simulink model "parameter_estimation"  (R2016a)
settings: Solver=VariableStepAuto  StartTime=0.0  StopTime=10.0  RelTol=1e-3
model workspace (MAT data in the model file):
  parameter_estimation_spesession : sldodialogs.data.SessionData (value not decoded)
undefined symbols (not defined in the file): Ts
settings Model: Creator=User  LastModifiedBy=User

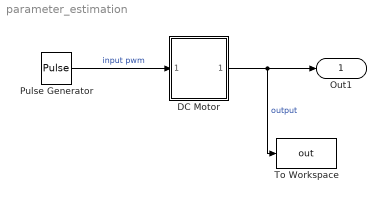
== system parameter_estimation ==
  DC Motor : Subsystem  mask(DC Motor){b=0.272617645619831, J=0.010032184368255, K=0.036496812786540, R=0.233319374033541, L=0.010005916298972}
      mask prompts: b "Damping:"; J "Inertia:"; K "Back EMF:"; R "Resistance:"; L "Inductance:"
      mask help: An ideal model of a DC Motor
      mask Help: This is <b>more elaborate<b> help.
      mask Display: image(imread('dcmotor.jpg'))
  Pulse Generator : DiscretePulseGenerator  PulseType=Time based  Period=0.1  PulseWidth=50  SampleTime=Ts  VectorParams1D=off
  To Workspace : ToWorkspace  VariableName=out  SampleTime=-1
  Out1 : Outport
  wires:
  DC Motor/1(Speed) -> To Workspace/1, Out1/1  "output"
  Pulse Generator/1 -> DC Motor/1(Voltage)  "input pwm"

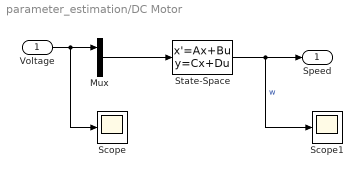
== system parameter_estimation/DC Motor ==
  Voltage : Inport
  Mux : Mux  Inputs=2
  Scope : Scope
  Scope1 : Scope
  State-Space : StateSpace  A=[-b/J K/J; -K/L -R/L]  B=[0 -1/J; 1/L 0]  C=[1 0]  D=[0 0]  X0=0
  Speed : Outport
  wires:
  State-Space/1 -> Scope1/1, Speed/1  "w"
  Voltage/1 -> Scope/1, Mux/1
  Mux/1 -> State-Space/1
